simulink model "FP_Solutions_Part_3_disturbance"  (R2022a)
settings: Solver=VariableStepAuto  StartTime=0.0  StopTime=tspan  FixedStep=10  RelTol=1e-8
model workspace (MATLAB code in the model file):
  | mu = 398601; % km
  | Re = 6378.137; %km
undefined symbols (not defined in the file): E_b_ECI_0, J, JD_0, m_b, q_b_ECI_0, r_ECI_0, sun_ECI, surfaceProperties, T_c, v_ECI_0, w_b_ECI_0
settings Model: Creator=emehiel  LastModifiedBy=emehiel
settings SolverCC: AlgebraicLoopSolver=TrustRegion
settings DebuggingCC: UnconnectedInputMsg=warning  UnconnectedOutputMsg=warning  UnconnectedLineMsg=warning  SFMachineParentedDataDiag=warning

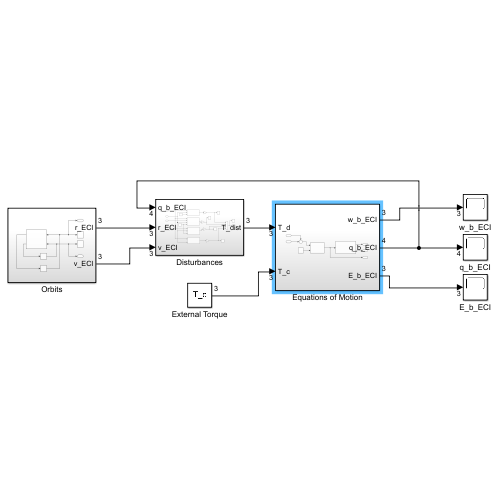
[thumbnail: Simulink's stored preview of the top-level diagram]
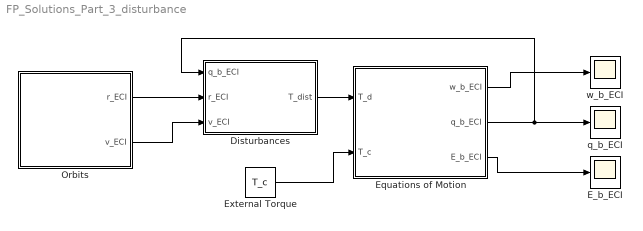
== system FP_Solutions_Part_3_disturbance ==
  Disturbances : Subsystem
  E_b_ECI : Scope
  Equations of Motion : Subsystem
  External Torque : Constant  Value=T_c
  Orbits : Subsystem
  q_b_ECI : Scope
  w_b_ECI : Scope
  wires:
  Orbits/1(r_ECI) -> Disturbances/2(r_ECI)
  Orbits/2(v_ECI) -> Disturbances/3(v_ECI)
  Equations of Motion/2(q_b_ECI) -> Disturbances/1(q_b_ECI), q_b_ECI/1
  Equations of Motion/1(w_b_ECI) -> w_b_ECI/1
  Disturbances/1(T_dist) -> Equations of Motion/1(T_d)
  Equations of Motion/3(E_b_ECI) -> E_b_ECI/1
  External Torque/1 -> Equations of Motion/2(T_c)

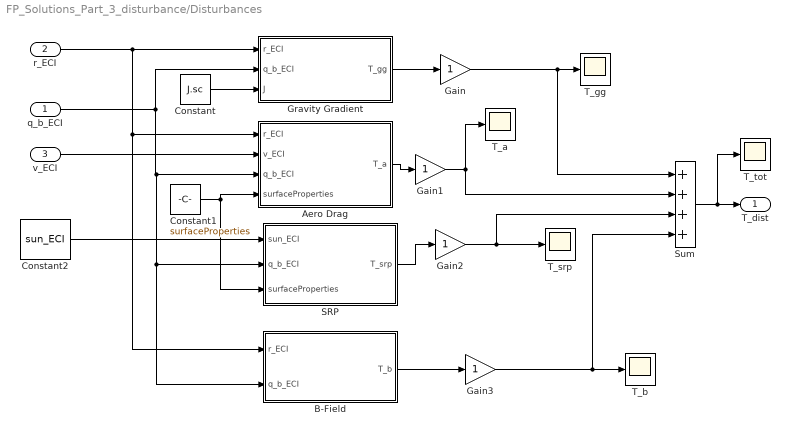
== system FP_Solutions_Part_3_disturbance/Disturbances ==
  q_b_ECI : Inport
  r_ECI : Inport  Port=2
  v_ECI : Inport  Port=3
  Aero Drag : MATLAB Function  TreatAsAtomicUnit=on
  B-Field : Subsystem
  Constant : Constant  Value=J.sc
  Constant1 : Constant  Value=surfaceProperties
  Constant2 : Constant  Value=sun_ECI
  Gain{,1..3} (4 alike) : Gain
  Gravity Gradient : MATLAB Function  TreatAsAtomicUnit=on
  SRP : MATLAB Function  TreatAsAtomicUnit=on
  Sum : Sum  Inputs=++++
  T_a : Scope
  T_b : Scope
  T_gg : Scope
  T_srp : Scope
  T_tot : Scope
  T_dist : Outport
  wires:
  Sum/1 -> T_tot/1, T_dist/1
  Aero Drag/1(T_a) -> Gain1/1
  Gravity Gradient/1(T_gg) -> Gain/1
  SRP/1(T_srp) -> Gain2/1
  Constant1/1 -> SRP/3(surfaceProperties), Aero Drag/4(surfaceProperties)
  v_ECI/1 -> Aero Drag/2(v_ECI)
  q_b_ECI/1 -> B-Field/2(q_b_ECI), SRP/2(q_b_ECI), Aero Drag/3(q_b_ECI), Gravity Gradient/2(q_b_ECI)
  Constant/1 -> Gravity Gradient/3(J)
  Constant2/1 -> SRP/1(sun_ECI)
  r_ECI/1 -> B-Field/1(r_ECI), Aero Drag/1(r_ECI), Gravity Gradient/1(r_ECI)
  B-Field/1(T_b) -> Gain3/1
  Gain/1 -> Sum/1, T_gg/1
  Gain1/1 -> Sum/2, T_a/1
  Gain2/1 -> Sum/3, T_srp/1
  Gain3/1 -> T_b/1, Sum/4

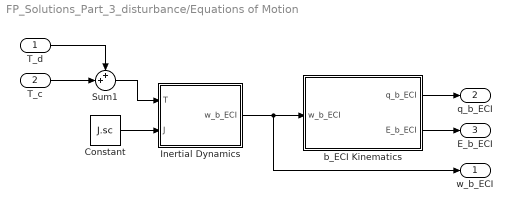
== system FP_Solutions_Part_3_disturbance/Equations of Motion ==
  T_d : Inport
  T_c : Inport  Port=2
  Constant : Constant  Value=J.sc
  Inertial Dynamics : Subsystem
  Sum1 : Sum  Inputs=++|
  b_ECI Kinematics : Subsystem
  w_b_ECI : Outport  VectorParamsAs1DForOutWhenUnconnected=off
  q_b_ECI : Outport  Port=2  VectorParamsAs1DForOutWhenUnconnected=off
  E_b_ECI : Outport  Port=3  VectorParamsAs1DForOutWhenUnconnected=off
  wires:
  b_ECI Kinematics/2(E_b_ECI) -> E_b_ECI/1
  Sum1/1 -> Inertial Dynamics/1(T)
  Constant/1 -> Inertial Dynamics/2(J)
  Inertial Dynamics/1(w_b_ECI) -> w_b_ECI/1, b_ECI Kinematics/1(w_b_ECI)
  T_d/1 -> Sum1/1
  T_c/1 -> Sum1/2
  b_ECI Kinematics/1(q_b_ECI) -> q_b_ECI/1

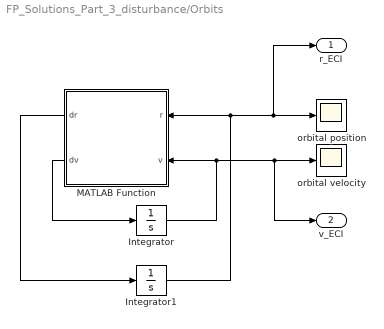
== system FP_Solutions_Part_3_disturbance/Orbits ==
  Integrator : Integrator  InitialCondition=v_ECI_0
  Integrator1 : Integrator  InitialCondition=r_ECI_0
  MATLAB Function : MATLAB Function  TreatAsAtomicUnit=on
  orbital position : Scope
  orbital velocity : Scope
  r_ECI : Outport  VectorParamsAs1DForOutWhenUnconnected=off
  v_ECI : Outport  Port=2  VectorParamsAs1DForOutWhenUnconnected=off
  wires:
  Integrator/1 -> v_ECI/1, orbital velocity/1, MATLAB Function/2(v)
  Integrator1/1 -> r_ECI/1, orbital position/1, MATLAB Function/1(r)
  MATLAB Function/1(dr) -> Integrator1/1
  MATLAB Function/2(dv) -> Integrator/1

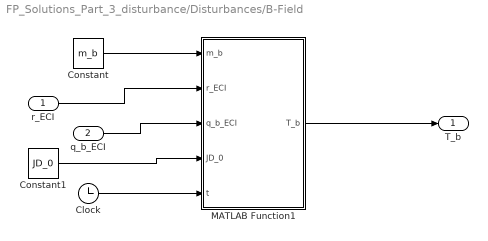
== system FP_Solutions_Part_3_disturbance/Disturbances/B-Field ==
  r_ECI : Inport
  q_b_ECI : Inport  Port=2
  Clock : Clock
  Constant : Constant  Value=m_b  VectorParams1D=off
  Constant1 : Constant  Value=JD_0
  MATLAB Function1 : MATLAB Function  TreatAsAtomicUnit=on
  T_b : Outport
  wires:
  q_b_ECI/1 -> MATLAB Function1/3(q_b_ECI)
  MATLAB Function1/1(T_b) -> T_b/1
  r_ECI/1 -> MATLAB Function1/2(r_ECI)
  Clock/1 -> MATLAB Function1/5(t)
  Constant1/1 -> MATLAB Function1/4(JD_0)
  Constant/1 -> MATLAB Function1/1(m_b)

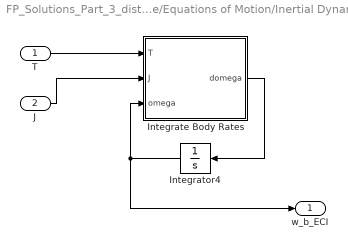
== system FP_Solutions_Part_3_disturbance/Equations of Motion/Inertial Dynamics ==
  T : Inport
  J : Inport  Port=2
  Integrate Body Rates : MATLAB Function  TreatAsAtomicUnit=on
  Integrator4 : Integrator  InitialCondition=w_b_ECI_0
  w_b_ECI : Outport  VectorParamsAs1DForOutWhenUnconnected=off
  wires:
  Integrate Body Rates/1(domega) -> Integrator4/1
  J/1 -> Integrate Body Rates/2(J)
  T/1 -> Integrate Body Rates/1(T)
  Integrator4/1 -> w_b_ECI/1, Integrate Body Rates/3(omega)

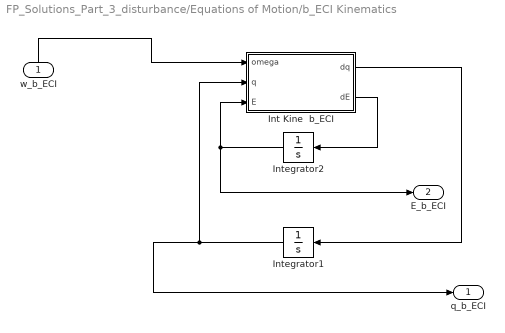
== system FP_Solutions_Part_3_disturbance/Equations of Motion/b_ECI Kinematics ==
  w_b_ECI : Inport
  Int Kine  b_ECI : MATLAB Function  TreatAsAtomicUnit=on
  Integrator1 : Integrator  InitialCondition=q_b_ECI_0
  Integrator2 : Integrator  InitialCondition=E_b_ECI_0
  q_b_ECI : Outport  VectorParamsAs1DForOutWhenUnconnected=off
  E_b_ECI : Outport  Port=2  VectorParamsAs1DForOutWhenUnconnected=off
  wires:
  w_b_ECI/1 -> Int Kine  b_ECI/1(omega)
  Int Kine  b_ECI/1(dq) -> Integrator1/1
  Int Kine  b_ECI/2(dE) -> Integrator2/1
  Integrator1/1 -> q_b_ECI/1, Int Kine  b_ECI/2(q)
  Integrator2/1 -> E_b_ECI/1, Int Kine  b_ECI/3(E)

== matlab function FP_Solutions_Part_3_disturbance/Equations of Motion/Inertial Dynamics/Integrate Body Rates ==
  data: T input; J input; omega input; domega output
function domega = dynamics(T, J, omega)
%#codegen

domega = J\(T - cross(omega, J*omega));

== matlab function FP_Solutions_Part_3_disturbance/Equations of Motion/b_ECI Kinematics/Int Kine  b_ECI ==
  data: omega input; q input; dq output; E input; dE output
function [dq,dE] = kinematics(omega, q, E)
%#codegen

% unpack quaternion

epsilon = q(1:3,1);
eta = q(4,1);

depsilon = 1/2*(eta*eye(3) + vect2cross(epsilon))*omega;
deta = -1/2*epsilon'*omega;

dq = [depsilon; deta];

LBI = 1/cos(E(2))*[cos(E(2)) sin(E(1))*sin(E(2))  cos(E(1))*sin(E(2));
                   0         cos(E(1))*cos(E(2)) -sin(E(1))*cos(E(2));
                   0         sin(E(1))            cos(E(1))];

dE = LBI*omega;

== matlab function FP_Solutions_Part_3_disturbance/Disturbances/Gravity Gradient ==
  data: r_ECI input; T_gg output; q_b_ECI input; J input
function T_gg = gg_torque(r_ECI, q_b_ECI, J)

mu = 398600; %km^3/s^2

r_b = quat2C(q_b_ECI)*r_ECI; %km

% Gravity Gradient Torque - don't need to convert mu or r
T_gg = 3*mu/norm(r_b)^5 * vect2cross(r_b)*J*(r_b);

== matlab function FP_Solutions_Part_3_disturbance/Disturbances/Aero Drag ==
  data: r_ECI input; v_ECI input; T_a output; q_b_ECI input; surfaceProperties input
function T_a = aero_drag_torque(r_ECI, v_ECI, q_b_ECI, surfaceProperties) 

v_b = quat2C(q_b_ECI)*v_ECI;
Cd = 2.1;
Re = 6378.137;

rho_0 = 3.614e-14;
H = 109.9;
h_0 = 700;
h = norm(r_ECI) - Re;
density = rho_0*exp(-(h - h_0)/H);
T_a = zeros([3,1]);

for i = 1:length(surfaceProperties)
    A = surfaceProperties(i,1);
    cp = surfaceProperties(i,2:4);
    n = surfaceProperties(i,5:7);
    wet = n*v_b/norm(v_b);
    if wet > 0
        A_wet = A*wet;
        v_b_hat = v_b/norm(v_b);
        F_a = -1/2*density*(norm(v_ECI)*1000)^2*Cd*A_wet*v_b_hat;
        T_a = T_a + cross(cp', F_a);
    end
end

== matlab function FP_Solutions_Part_3_disturbance/Disturbances/SRP ==
  data: sun_ECI input; T_srp output; q_b_ECI input; surfaceProperties input
function T_srp  = SPR_torque(sun_ECI, q_b_ECI, surfaceProperties)

p_sun = 4.5e-6; %N/m

sun_b = quat2C(q_b_ECI)*sun_ECI;
T_srp = zeros([3,1]);
%rho_sum = zeros([3,1]);
% Solar Radiation Pressure
for i = 1:length(surfaceProperties)
    A = surfaceProperties(i,1);
    cp = surfaceProperties(i,2:4);
    n = surfaceProperties(i,5:7);
    wet = n*sun_b/norm(sun_b);
    if wet > 0
        A_wet = A*wet;
        F_srp = p_sun*A_wet*sun_b;
        T_srp = T_srp + cross(cp', F_srp);
        %rho_sum = rho_sum + rho';
    end
end

== matlab function FP_Solutions_Part_3_disturbance/Orbits/MATLAB Function ==
  data: r input; dr output; v input; dv output
function [dr,dv] = orbitalDynamics(r, v)
%#codegen

mu = 398600; % km^3/s^2

dr = v;
dv = -mu*r/norm(r)^3;

== matlab function FP_Solutions_Part_3_disturbance/Disturbances/B-Field/MATLAB Function1 ==
  data: m_b input; r_ECI input; q_b_ECI input; T_b output; JD_0 input; t input
function T_b = WMM(m_b, r_ECI, q_b_ECI, JD_0, t)

% DGRF 2020 
a = 6371.2; %km
g_11 = -1450.9; %nT
h_11 = 4652.5; %nT
g_10 = -29404.8; %nT
m_ECEF = a^3*[g_11; h_11; g_10];

m_ECEF = m_ECEF*1e-9*1000^3; %convert km^3*nT to m^3*T

r_ECI = r_ECI*1000; % convert km to m
r = norm(r_ECI);
JD = JD_0 + t/(24*3600);
[lat, long, alt, gst] = eci2lla2(JD, r_ECI);

m_ECI = Cz(-long*pi/180) * m_ECEF;

B_ECI = (3*m_ECI'*r_ECI*r_ECI - r^2*m_ECI)/r^5;

C_b_ECI = quat2C(q_b_ECI);

B_b = C_b_ECI*B_ECI;

T_b = vect2cross(m_b)*B_b;
